simulink subsystem "Object"  (R2023a)
settings: Solver=VariableStepAuto  StartTime=0.0  StopTime=10.0  RelTol=1e-3
undefined symbols (not defined in the file): Azimuth_initial_angle, Elevation_initial_angle, J_azimuth, J_elevation
settings Model: Creator=ycheb  LastModifiedBy=ycheb

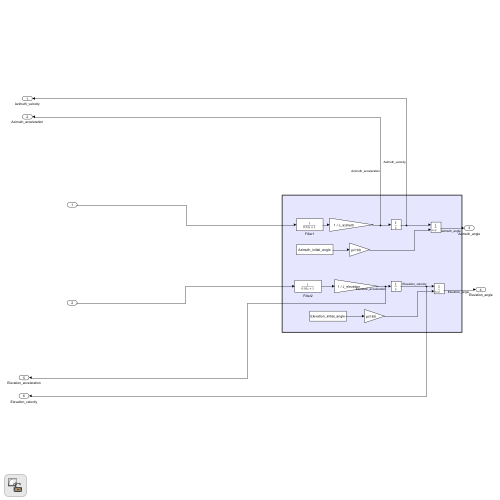
[thumbnail: Simulink's stored preview of the top-level diagram]
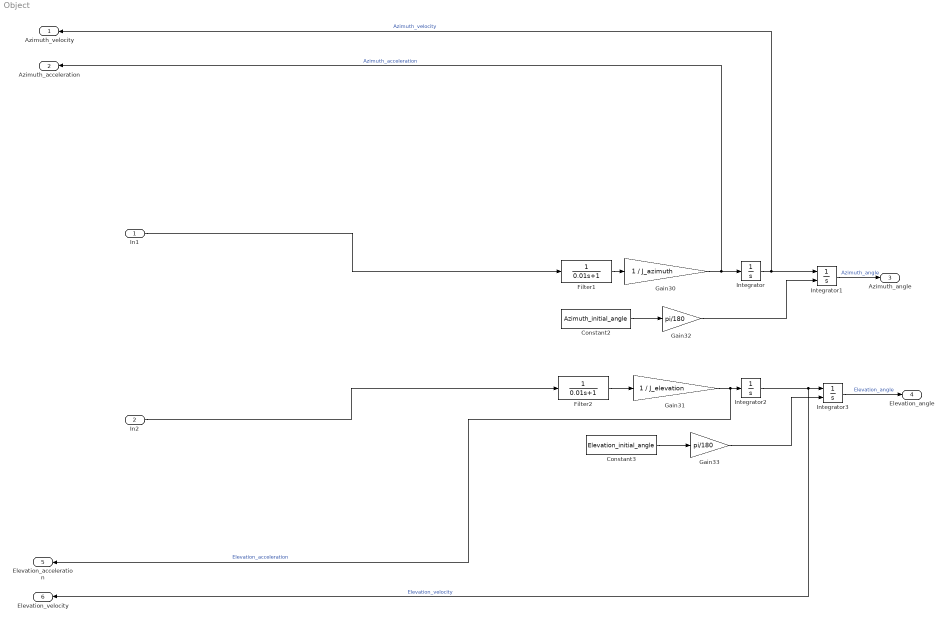
== system Object ==
  In1 : Inport
  In2 : Inport  Port=2
  Constant2 : Constant  Value=Azimuth_initial_angle
  Constant3 : Constant  Value=Elevation_initial_angle
  Filter1 : TransferFcn  Denominator=[0.01 1]
  Filter2 : TransferFcn  Denominator=[0.01 1]
  Gain30 : Gain  Gain=1 / J_azimuth
  Gain31 : Gain  Gain=1 / J_elevation
  Gain32 : Gain  Gain=pi/180
  Gain33 : Gain  Gain=pi/180
  Integrator : Integrator
  Integrator1 : Integrator  InitialConditionSource=external
  Integrator2 : Integrator
  Integrator3 : Integrator  InitialConditionSource=external
  Azimuth_velocity : Outport
  Azimuth_acceleration : Outport  Port=2
  Azimuth_angle : Outport  Port=3
  Elevation_angle : Outport  Port=4
  Elevation_acceleration : Outport  Port=5
  Elevation_velocity : Outport  Port=6
  wires:
  Filter1/1 -> Gain30/1
  Gain33/1 -> Integrator3/2
  Integrator2/1 -> Integrator3/1, Elevation_velocity/1  "Elevation_velocity"
  Gain30/1 -> Integrator/1, Azimuth_acceleration/1  "Azimuth_acceleration"
  Gain32/1 -> Integrator1/2
  Constant3/1 -> Gain33/1
  Gain31/1 -> Integrator2/1, Elevation_acceleration/1  "Elevation_acceleration"
  In2/1 -> Filter2/1
  Filter2/1 -> Gain31/1
  Constant2/1 -> Gain32/1
  Integrator/1 -> Integrator1/1, Azimuth_velocity/1  "Azimuth_velocity"
  In1/1 -> Filter1/1
  Integrator1/1 -> Azimuth_angle/1  "Azimuth_angle"
  Integrator3/1 -> Elevation_angle/1  "Elevation_angle"
